simulink model "discrete_bug"  (Simulink 7.1)
settings: Solver=ode45  StartTime=0.0  StopTime=10.0  RelTol=1e-3
settings Model: Creator=kamimoto  LastModifiedBy=toida
settings DebuggingCC: SaveWithParameterizedLinksMsg=none
settings GRTTargetCC: TargetFcnLib=ansi_tfl_tmw.mat

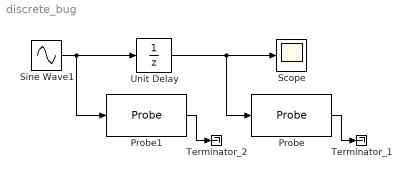
== system discrete_bug ==
  Probe : Probe  ProbeWidth=off  ProbeComplexSignal=off
  Probe1 : Probe  ProbeWidth=off  ProbeComplexSignal=off
  Scope : Scope
      settings: TimeRange=10  YMin=-1  YMax=1
  Sine Wave1 : Sin  SampleTime=0.1
  Terminator_1 : Terminator
  Terminator_2 : Terminator
  Unit Delay : UnitDelay
  wires:
  Sine Wave1/1 -> Unit Delay/1, Probe1/1
  Unit Delay/1 -> Scope/1, Probe/1
  Probe/1 -> Terminator_1/1
  Probe1/1 -> Terminator_2/1
